simulink model "practico_1_linearization"  (R2021b)
settings: Solver=VariableStepAuto  StartTime=0.0  StopTime=60.0  RelTol=1e-3
values from neighbouring files (symbols this model uses):
  A_d = exp(dfdh_eval*Ts)    [p1_code.m]
  B_d = dfdh_eval^(-1) * (A_d-1) * dfdk_eval    [p1_code.m]
  dfdh_eval = double(vpa(subs(dfdh, [h, k], [h_bar, k_bar])))    [p1_code.m]
  dfdk_eval = double(vpa(subs(dfdk, [h, k], [h_bar, k_bar])))    [p1_code.m]
  h_bar = 0.2    [p1_code.m]
  k_bar = F_in / (a*sqrt(2*9.81*h_bar))    [p1_code.m]
  k_list = [0.05, 0.15, 0.30, 0.50, 0.90]    [p1_code.m]
  Ts = 1    [p1_code.m]
undefined symbols (not defined in the file or in its folder): den, num, T
settings Model: Creator=trulscarlson  LastModifiedBy=trulscarlson

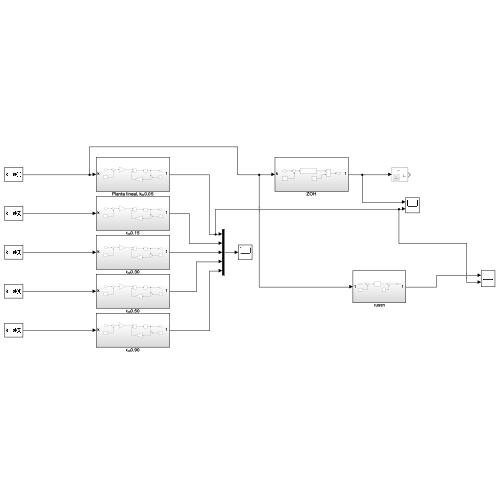
[thumbnail: Simulink's stored preview of the top-level diagram]
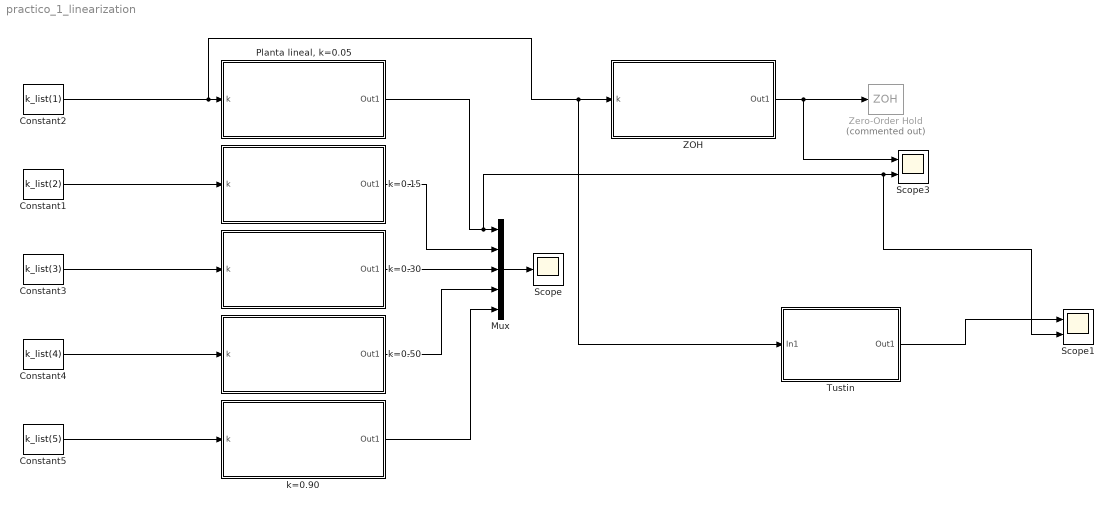
== system practico_1_linearization ==
  Constant1 : Constant  Value=k_list(2)
  Constant2 : Constant  Value=k_list(1)
  Constant3 : Constant  Value=k_list(3)
  Constant4 : Constant  Value=k_list(4)
  Constant5 : Constant  Value=k_list(5)
  Mux : Mux  Inputs=5
  "Planta lineal, k=0.05" : Subsystem
  Scope : Scope
  Scope1 : Scope  NumInputPorts=2
  Scope3 : Scope  NumInputPorts=2
  Tustin : Subsystem
  ZOH : Subsystem
  Zero-Order Hold : ZeroOrderHold  Commented=on  SampleTime=T
  k=0.15 : Subsystem
  k=0.30 : Subsystem
  k=0.50 : Subsystem
  k=0.90 : Subsystem
  wires:
  Constant2/1 -> Tustin/1(In1), ZOH/1(k), "Planta lineal, k=0.05"/1(k)
  Constant3/1 -> k=0.30/1(k)
  Constant4/1 -> k=0.50/1(k)
  Constant5/1 -> k=0.90/1(k)
  Mux/1 -> Scope/1
  "Planta lineal, k=0.05"/1(Out1) -> Scope1/2, Scope3/2, Mux/1
  k=0.30/1(Out1) -> Mux/3
  k=0.50/1(Out1) -> Mux/4
  k=0.90/1(Out1) -> Mux/5
  ZOH/1(Out1) -> Scope3/1, Zero-Order Hold/1
  Tustin/1(Out1) -> Scope1/1
  Constant1/1 -> k=0.15/1(k)
  k=0.15/1(Out1) -> Mux/2

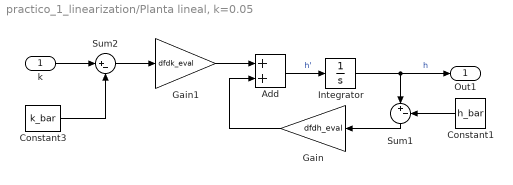
== system practico_1_linearization/Planta lineal, k=0.05 ==
  k : Inport
  Add : Sum
  Constant1 : Constant  Value=h_bar
  Constant3 : Constant  Value=k_bar
  Gain : Gain  Gain=dfdh_eval
  Gain1 : Gain  Gain=dfdk_eval
  Integrator : Integrator  InitialCondition=h_bar
  Sum1 : Sum  Inputs=|+-
  Sum2 : Sum  Inputs=|+-
  Out1 : Outport
  wires:
  k/1 -> Sum2/1
  Gain1/1 -> Add/1
  Add/1 -> Integrator/1  "h'"
  Constant3/1 -> Sum2/2
  Integrator/1 -> Out1/1, Sum1/1  "h"
  Sum2/1 -> Gain1/1
  Sum1/1 -> Gain/1
  Gain/1 -> Add/2
  Constant1/1 -> Sum1/2

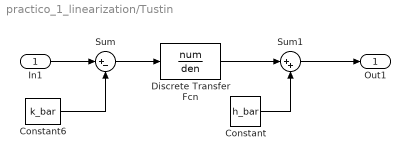
== system practico_1_linearization/Tustin ==
  In1 : Inport
  Constant : Constant  Value=h_bar
  Constant6 : Constant  Value=k_bar
  Discrete Transfer Fcn : DiscreteTransferFcn  Numerator=num  Denominator=den  SampleTime=2
  Sum : Sum  Inputs=|+-
  Sum1 : Sum  Inputs=|++
  Out1 : Outport
  wires:
  Sum1/1 -> Out1/1
  Constant/1 -> Sum1/2
  Constant6/1 -> Sum/2
  Sum/1 -> Discrete Transfer Fcn/1
  Discrete Transfer Fcn/1 -> Sum1/1
  In1/1 -> Sum/1

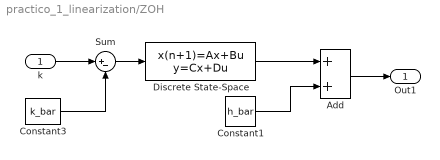
== system practico_1_linearization/ZOH ==
  k : Inport
  Add : Sum
  Constant1 : Constant  Value=h_bar
  Constant3 : Constant  Value=k_bar
  Discrete State-Space : DiscreteStateSpace  A=A_d  B=B_d  D=0  SampleTime=Ts
  Sum : Sum  Inputs=|+-
  Out1 : Outport
  wires:
  k/1 -> Sum/1
  Constant3/1 -> Sum/2
  Sum/1 -> Discrete State-Space/1
  Constant1/1 -> Add/2
  Discrete State-Space/1 -> Add/1
  Add/1 -> Out1/1

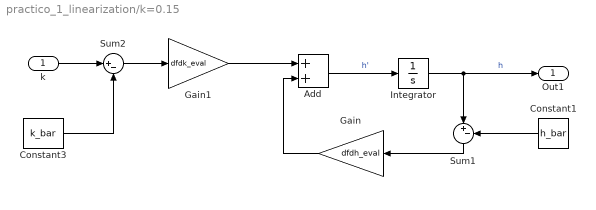
== system practico_1_linearization/k=0.15 ==
  k : Inport
  Add : Sum
  Constant1 : Constant  Value=h_bar
  Constant3 : Constant  Value=k_bar
  Gain : Gain  Gain=dfdh_eval
  Gain1 : Gain  Gain=dfdk_eval
  Integrator : Integrator  InitialCondition=h_bar
  Sum1 : Sum  Inputs=|+-
  Sum2 : Sum  Inputs=|+-
  Out1 : Outport
  wires:
  k/1 -> Sum2/1
  Gain1/1 -> Add/1
  Add/1 -> Integrator/1  "h'"
  Constant3/1 -> Sum2/2
  Integrator/1 -> Out1/1, Sum1/1  "h"
  Sum2/1 -> Gain1/1
  Sum1/1 -> Gain/1
  Gain/1 -> Add/2
  Constant1/1 -> Sum1/2

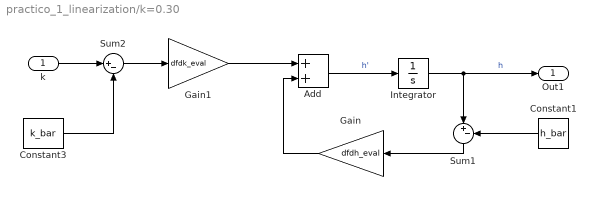
== system practico_1_linearization/k=0.30 ==
  k : Inport
  Add : Sum
  Constant1 : Constant  Value=h_bar
  Constant3 : Constant  Value=k_bar
  Gain : Gain  Gain=dfdh_eval
  Gain1 : Gain  Gain=dfdk_eval
  Integrator : Integrator  InitialCondition=h_bar
  Sum1 : Sum  Inputs=|+-
  Sum2 : Sum  Inputs=|+-
  Out1 : Outport
  wires:
  k/1 -> Sum2/1
  Gain1/1 -> Add/1
  Add/1 -> Integrator/1  "h'"
  Constant3/1 -> Sum2/2
  Integrator/1 -> Out1/1, Sum1/1  "h"
  Sum2/1 -> Gain1/1
  Sum1/1 -> Gain/1
  Gain/1 -> Add/2
  Constant1/1 -> Sum1/2

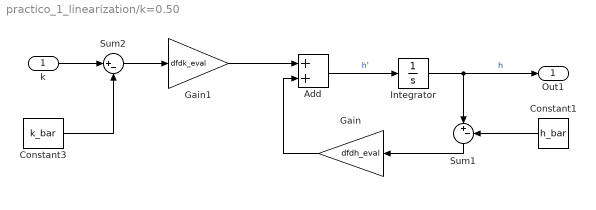
== system practico_1_linearization/k=0.50 ==
  k : Inport
  Add : Sum
  Constant1 : Constant  Value=h_bar
  Constant3 : Constant  Value=k_bar
  Gain : Gain  Gain=dfdh_eval
  Gain1 : Gain  Gain=dfdk_eval
  Integrator : Integrator  InitialCondition=h_bar
  Sum1 : Sum  Inputs=|+-
  Sum2 : Sum  Inputs=|+-
  Out1 : Outport
  wires:
  k/1 -> Sum2/1
  Gain1/1 -> Add/1
  Add/1 -> Integrator/1  "h'"
  Constant3/1 -> Sum2/2
  Integrator/1 -> Out1/1, Sum1/1  "h"
  Sum2/1 -> Gain1/1
  Sum1/1 -> Gain/1
  Gain/1 -> Add/2
  Constant1/1 -> Sum1/2

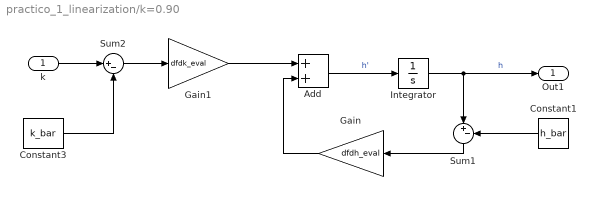
== system practico_1_linearization/k=0.90 ==
  k : Inport
  Add : Sum
  Constant1 : Constant  Value=h_bar
  Constant3 : Constant  Value=k_bar
  Gain : Gain  Gain=dfdh_eval
  Gain1 : Gain  Gain=dfdk_eval
  Integrator : Integrator  InitialCondition=h_bar
  Sum1 : Sum  Inputs=|+-
  Sum2 : Sum  Inputs=|+-
  Out1 : Outport
  wires:
  k/1 -> Sum2/1
  Gain1/1 -> Add/1
  Add/1 -> Integrator/1  "h'"
  Constant3/1 -> Sum2/2
  Integrator/1 -> Out1/1, Sum1/1  "h"
  Sum2/1 -> Gain1/1
  Sum1/1 -> Gain/1
  Gain/1 -> Add/2
  Constant1/1 -> Sum1/2
